simulink model "assi_flash_logic"  (R2025a)
settings: Solver=VariableStepAuto  StartTime=0.0  StopTime=10.0  RelTol=1e-3
model workspace (MAT data in the model file):
  FLASH_DUR = Simulink.NumericType
  FLASH_DUR.DataTypeMode = 'Double'
  FLASH_DUR.SignednessBool = 1
  FLASH_DUR.WordLength = 64
  FLASH_DUR.FixedExponent = 0
  FLASH_DUR.SlopeAdjustmentFactor = 1
  FLASH_DUR.Bias = 0
  FLASH_DUR.DataTypeOverride = 'Inherit'
  FLASH_DUR.IsAlias = 0
  FLASH_DUR.DataScope = 'Auto'
libraries: simulink x1
settings Model: Creator=Imade  LastModifiedBy=Imade

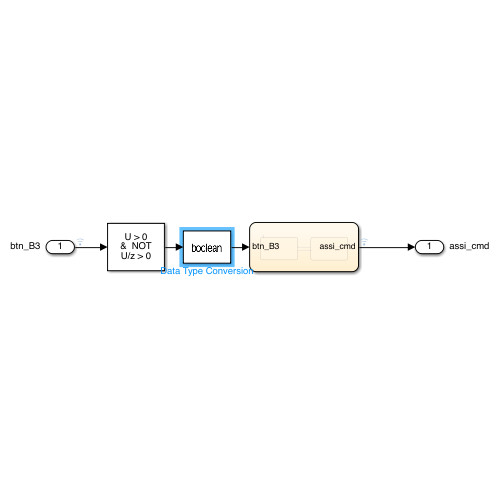
[thumbnail: Simulink's stored preview of the top-level diagram]
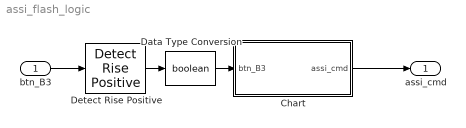
== system assi_flash_logic ==
  btn_B3 : Inport
  Chart : Stateflow chart  TreatAsAtomicUnit=on
  Data Type Conversion : DataTypeConversion  OutDataTypeStr=boolean  SaturateOnIntegerOverflow=off  RndMeth=Floor
  Detect Rise Positive : simulink/Logic and Bit Operations/Detect Rise Positive  vinit=0  OutDataTypeStr=boolean
  assi_cmd : Outport
  wires:
  Chart/1(assi_cmd) -> assi_cmd/1
  btn_B3/1 -> Detect Rise Positive/1
  Detect Rise Positive/1 -> Data Type Conversion/1
  Data Type Conversion/1 -> Chart/1(btn_B3)

== stateflow chart assi_flash_logic/Chart ==
  settings: updateMethod=DISCRETE  sampleTime=0.001
  state ACTIVE
    during:
    assi_cmd = true;
  state IDLE
    during:
    assi_cmd = false;
  (default) -> IDLE
  ACTIVE -> IDLE : [after(FLASH_DUR, sec)]
  IDLE -> ACTIVE : [btn_B3]
  data: btn_B3 input; assi_cmd output; FLASH_DUR constant double =0.5
